simulink model "zero_to_hero_sect11_plant"  (R2023a)
settings: Solver=VariableStepAuto  StartTime=0.0  StopTime=simtime  MaxStep=0.01  RelTol=1e-3
values from neighbouring files (symbols this model uses):
  b = 50    [zero_to_hero_sect10_script.m]    (also in zero_to_hero_sect1to5_script.m = 0.1; zero_to_hero_sect7to8_script.m = 10)
undefined symbols (not defined in the file or in its folder): J_Mo, K_m, L, R, U_e
settings Model: Creator=fycce  LastModifiedBy=fycce
settings DataIOCC: SaveOutput=off  SaveTime=off  ReturnWorkspaceOutputs=off

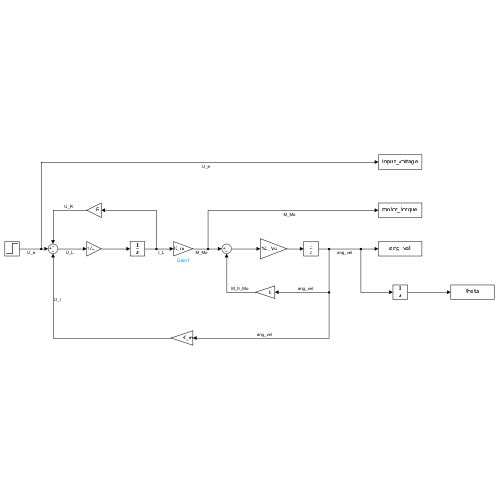
[thumbnail: Simulink's stored preview of the top-level diagram]
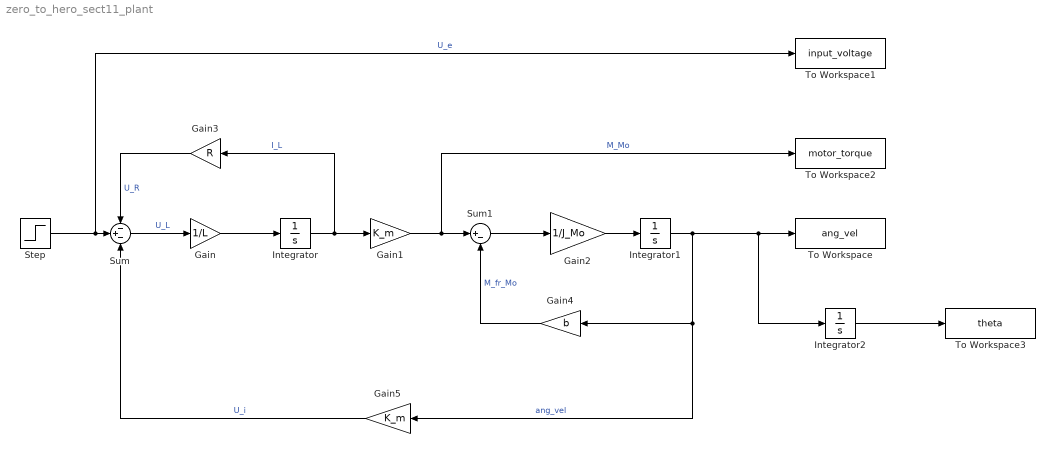
== system zero_to_hero_sect11_plant ==
  Gain : Gain  Gain=1/L
  Gain1 : Gain  Gain=K_m
  Gain2 : Gain  Gain=1/J_Mo
  Gain3 : Gain  Gain=R
  Gain4 : Gain  Gain=b
  Gain5 : Gain  Gain=K_m
  Integrator : Integrator
  Integrator1 : Integrator
  Integrator2 : Integrator
  Step : Step  Time=U_e  SampleTime=0
  Sum : Sum  Inputs=-+-
  Sum1 : Sum  Inputs=|+-
  To Workspace : ToWorkspace  VariableName=ang_vel  SaveFormat=Timeseries  SampleTime=-1
  To Workspace1 : ToWorkspace  VariableName=input_voltage  SaveFormat=Timeseries  SampleTime=-1
  To Workspace2 : ToWorkspace  VariableName=motor_torque  SaveFormat=Timeseries  SampleTime=-1
  To Workspace3 : ToWorkspace  VariableName=theta  SaveFormat=Timeseries  SampleTime=-1
  wires:
  Step/1 -> To Workspace1/1, Sum/2  "U_e"
  Sum/1 -> Gain/1  "U_L"
  Gain/1 -> Integrator/1
  Integrator/1 -> Gain3/1, Gain1/1  "I_L"
  Gain1/1 -> To Workspace2/1, Sum1/1  "M_Mo"
  Sum1/1 -> Gain2/1
  Gain2/1 -> Integrator1/1
  Integrator1/1 -> Gain4/1, Gain5/1, To Workspace/1, Integrator2/1  "ang_vel"
  Gain3/1 -> Sum/1  "U_R"
  Gain4/1 -> Sum1/2  "M_fr_Mo"
  Gain5/1 -> Sum/3  "U_i"
  Integrator2/1 -> To Workspace3/1
